simulink model "antiwindup"  (R2015a)
settings: Solver=ode45  StartTime=0.0  StopTime=10.0  RelTol=1e-3
libraries: simulink x1
settings Model: Creator=Teme  LastModifiedBy=Teme
settings RTWCC: Toolchain=Clang v3.1 | gmake (64-bit Mac)

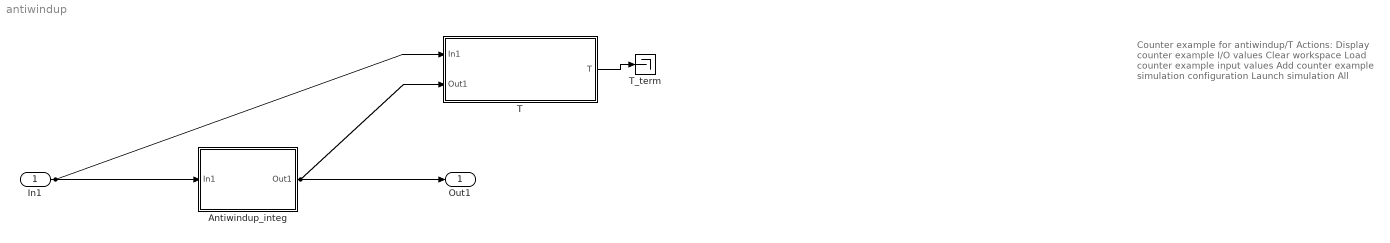
== system antiwindup ==
  note: Counter example for antiwindup/T
      | Actions:
      | Display counter example I/O values
      | Clear workspace
      | Load counter example input values
      | Add counter example simulation configuration
      | Launch simulation
      | All
  In1 : Inport
  Antiwindup_integ : Subsystem
  T : Subsystem  TreatAsAtomicUnit=on  mask(Observer){AnnotationType=ensures, ObserverType=[]}
      mask prompts: AnnotationType "Type of annotation (pre/post...)"; ObserverType "Observer type"
      mask help:
      | Set an observer for the system.
      | The annotation type parameter sets the type of observer:
      | - requires : pre-condition
      | - ensures : post-condition
      | - assert : an assertion
      | - observer : the observer computes a special type of properties
      mask TypeOptions AnnotationType: ensures | requires | assert | observer
      mask Callback AnnotationType:
      | paramStr = get_param(gcb, 'MaskValues');
      | if strcmp(paramStr{1}(1),'o')
      | set_param(gcb,'MaskVisibilities',{'on';'on'});
      | paramStr{2} = 'ellipsoid';
      | set_param(gcb,'MaskValues',paramStr);
      | else
      | set_param(gcb,'MaskVisibilities',{'on';'off'});
      | end
      | clear paramStr;
      mask Callback ObserverType:
      | paramStr = get_param(gcb, 'MaskValues');
      | if strcmp(paramStr{1}(1),'o')
      | set_param(gcb,'MaskVisibilities',{'on';'on'});
      | paramStr{2} = 'ellipsoid';
      | set_param(gcb,'MaskValues',paramStr);
      | else
      | set_param(gcb,'MaskVisibilities',{'on';'off'});
      | end
      | clear paramStr;
      mask Display:
      | color('black')
      | text(0.5, 0.5, ['Property: ''' get_param(gcb,'name') ''''], 'horizontalAlignment', 'center');
      | text(0.99, 0.03, '{\bf\fontsize{12}CEX}', 'hor', 'right', 'ver', 'bottom', 'texmode', 'on');
  T_term : Terminator
  Out1 : Outport
  wires:
  In1/1 -> Antiwindup_integ/1(In1), T/1(In1)
  Antiwindup_integ/1(Out1) -> Out1/1, T/2(Out1)
  T/1(T) -> T_term/1

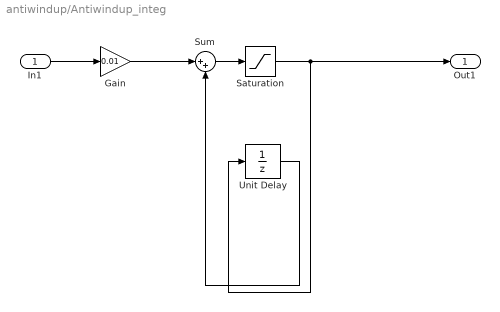
== system antiwindup/Antiwindup_integ ==
  In1 : Inport
  Gain : Gain  Gain=0.01
  Saturation : Saturate
  Sum : Sum  Inputs=|++
  Unit Delay : UnitDelay  SampleTime=-1
  Out1 : Outport
  wires:
  Sum/1 -> Saturation/1
  Gain/1 -> Sum/1
  Saturation/1 -> Unit Delay/1, Out1/1
  Unit Delay/1 -> Sum/2
  In1/1 -> Gain/1

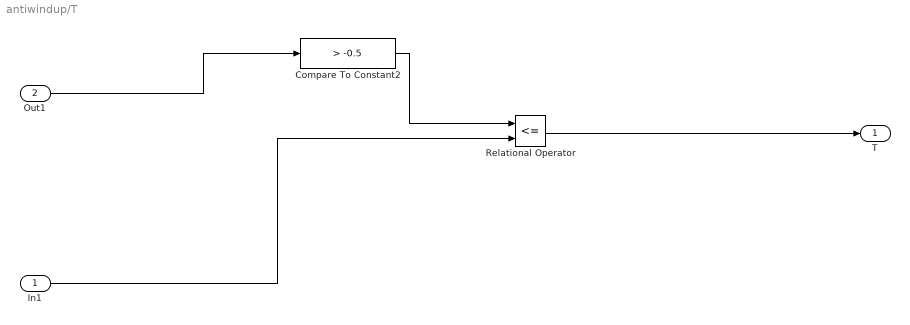
== system antiwindup/T ==
  In1 : Inport
  Out1 : Inport  Port=2
  Compare To Constant2 : simulink/Logic and Bit Operations/Compare To Constant  relop=>  const=-0.5  OutDataTypeStr=boolean
  Relational Operator : RelationalOperator  Operator=<=  OutDataTypeStr=boolean
  T : Outport
  wires:
  Out1/1 -> Compare To Constant2/1
  In1/1 -> Relational Operator/2
  Relational Operator/1 -> T/1
  Compare To Constant2/1 -> Relational Operator/1
